simulink model "computeFRI_fromSensors"  (Simulink 8.3)
settings: Solver=FixedStepDiscrete  StartTime=0.0  StopTime=inf  FixedStep=0.01  RelTol=1e-3
libraries: WBCLibrary x2
settings Model: Creator=jorhabib  LastModifiedBy=jorhabib
settings DataIOCC: SignalLoggingSaveFormat=Dataset
settings DebuggingCC: UnderspecifiedInitializationDetection=Simplified  StateNameClashWarn=none
settings GRTTargetCC: CombineOutputUpdateFcns=on  GRTInterface=off

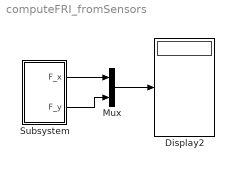
== system computeFRI_fromSensors ==
  Display2 : Display
  Mux : Mux  Inputs=2
  Subsystem : Subsystem  mask{robotName='iCubGenova01', localName='friFromModel', Ts=0.01}
      mask prompts: robotName "Robot name"; localName "Local name"
  wires:
  Subsystem/1(F_x) -> Mux/1
  Subsystem/2(F_y) -> Mux/2
  Mux/1 -> Display2/1

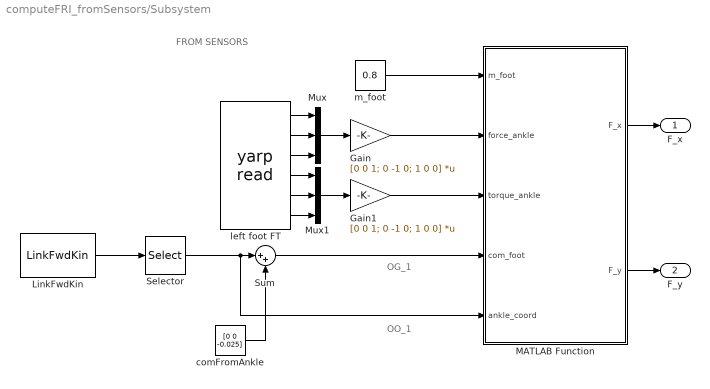
== system computeFRI_fromSensors/Subsystem ==
  note: FROM SENSORS
  note: OG_1
  note: OO_1
  Gain : Gain  Gain=[0 0 1; 0 -1 0; 1 0 0]  Multiplication=Matrix(K*u)  SampleTime=Ts
  Gain1 : Gain  Gain=[0 0 1; 0 -1 0; 1 0 0]  Multiplication=Matrix(K*u)  SampleTime=Ts
  LinkFwdKin : WBCLibrary/wholeBodyModel/Forward Kinematics/LinkFwdKin  robotname=robotName  localname=localName  link=l_ankle_1
  MATLAB Function : MATLAB Function  TreatAsAtomicUnit=on
  Mux : Mux  Inputs=3
  Mux1 : Mux  Inputs=3
  Selector : Selector  InputPortWidth=7  Indices=[1:3]
  Sum : Sum  Inputs=|++  SampleTime=Ts
  "comFromAnkle " : Constant  Value=[0 0 -0.025]  SampleTime=Ts
  left foot FT : WBCLibrary/Utilities/yarp read  from='/wbdt/joint_ankle_cartesian_wrench:o'  to='...'  num=6
  m_foot : Constant  Value=0.8  SampleTime=Ts
  F_x : Outport
  F_y : Outport  Port=2
  wires:
  m_foot/1 -> MATLAB Function/1(m_foot)
  left foot FT/3 -> Mux/3
  Mux/1 -> Gain/1
  Mux1/1 -> Gain1/1
  Selector/1 -> MATLAB Function/5(ankle_coord), Sum/1
  left foot FT/1 -> Mux/1
  Gain1/1 -> MATLAB Function/3(torque_ankle)
  left foot FT/2 -> Mux/2
  Gain/1 -> MATLAB Function/2(force_ankle)
  left foot FT/5 -> Mux1/2
  left foot FT/6 -> Mux1/3
  "comFromAnkle "/1 -> Sum/2
  Sum/1 -> MATLAB Function/4(com_foot)
  LinkFwdKin/1 -> Selector/1
  MATLAB Function/1(F_x) -> F_x/1
  left foot FT/4 -> Mux1/1
  MATLAB Function/2(F_y) -> F_y/1

== matlab function Subsystem/MATLAB Function ==
  data: F_x output double; m_foot input double; force_ankle input double; torque_ankle input double; com_foot input double; ankle_coord input double; F_y output double
function [F_x, F_y] = SOF(m_foot, force_ankle, torque_ankle,com_foot, ankle_coord)
%#codegen

grav = [0 0 9.8]';

grav = [0 0 -9.8]';
g_z = abs(grav(3));

F_x = (-torque_ankle(2) - ankle_coord(3)*force_ankle(1) + ankle_coord(1)*force_ankle(3) + m_foot*g_z*com_foot(1)) / (m_foot*g_z + force_ankle(3));
F_y = ( torque_ankle(1) - ankle_coord(3)*force_ankle(2) + ankle_coord(2)*force_ankle(3) + m_foot*g_z*com_foot(2)) / (m_foot*g_z + force_ankle(3));
